simulink model "bipedal_robot_CTRL2"  (R2020b)
settings: Solver=ode23  StartTime=0.0  StopTime=Tsim  MaxStep=0.01  RelTol=1e-3  AbsTol=1e-3  EnableMultiTasking=on
values from neighbouring files (symbols this model uses):
  g = 9.80665    [bipedal.m]
  Tfil = Ts*10    (= 0.01)    [bipedal.m]
  total_mass = mlist(1) + ll_mass + rl_mass    [bipedal.m]
  Ts = 1/fs    (= 0.001)    [bipedal.m]
undefined symbols (not defined in the file or in its folder): Base, ctrl_cfg_rem, Fdist, LefAnklePitch, LefAnkleRoll, LefHipPitch, LefHipRoll, LefHipYaw, LefKnee, pg_traj, RigAnklePitch, RigAnkleRoll, RigHipPitch, RigHipRoll, RigHipYaw, RigKnee, sim_floor, Tdist, VAR_DIST, X, Y, Z
libraries: sm_lib x56, biped_lib x39, nesl_utility x18, simulink x3, Contact_Forces_Lib x2, robotmaniplib x1
(part 4 of 4)

== matlab function bipedal_robot_CTRL2/Controller Version 2/Compute torques/Error computation ==
  data: ctrl_cfg input; q_ref input; qp_ref input; qL input; errL output; qR input; errR output; errL_p output; errR_p output; intL output; intR output; qLp input; qRp input
function [errL, errR, errL_p, errR_p, intL, intR] = fcn(ctrl_cfg, q_ref, qp_ref, qL, qR, qLp, qRp)
persistent init errL_int errR_int;
if isempty(init)
   init = 1;
   errL_int = zeros(6,1);
   errR_int = zeros(6,1);
end

dt = ctrl_cfg.par.Ts;

% reference positions
qL_ref = q_ref(1:end/2);
qR_ref = q_ref(end/2+1:end);
% reference velocities
qLp_ref = qp_ref(1:end/2);
qRp_ref = qp_ref(end/2+1:end);


% measured positions
qL_m = qL;
qR_m = qR;
% measured velocities
qLp_m = qLp;
qRp_m = qRp;

% position errors
errL = qL_ref-qL_m;
errR = qR_ref-qR_m;

% integral term
errL_int = errL_int + dt * errL;
intL = errL_int;
errR_int = errR_int + dt * errR;
intR = errR_int;

% velocity errors
errL_p = qLp_ref-qLp_m;
errR_p = qRp_ref-qRp_m;

== matlab function bipedal_robot_CTRL2/Controller Version 2/Inverse kinematics optimization/Fmincon Ikine (Matlab)/Full body IKine solver ==
  data: FSM input; ctrl_cfg input; meas input; q_ref output; cmds input; Jlist input; phase input; cont_data input; qp_ref output; q_ini input; qp_ini input; FmL input; FmR input
function [q_ref,qp_ref] = fcn(FSM, ctrl_cfg, meas, cmds, Jlist, phase, cont_data, q_ini, qp_ini, FmL,FmR)
% check if ikine is activated
if FSM.ikine
    test_type = ctrl_cfg.fsm.test_type;
    
    if test_type==-1
        [q_ref,qp_ref] = ikine_step_iktest(meas, cmds, q_ini, qp_ini, Jlist, ctrl_cfg, phase, cont_data);
    else
        [q_ref,qp_ref] = ikine_step2(meas, cmds, q_ini, qp_ini, Jlist, ctrl_cfg, phase, cont_data);
    end
    
    active_FT_ctrl = 0;
    Ts = ctrl_cfg.par.Ts;
    [q_ref,qp_ref] = foot_tilt_ctrl2(FmL, FmR, q_ref, qp_ref, Ts, active_FT_ctrl);
    
    
else
    q_ref = q_ini;
    qp_ref = qp_ini;
end

== matlab function bipedal_robot_CTRL2/Controller Version 2/Finite state machine ==
  data: time input; FSM output Bus: FSM_bus; ctrl_cfg input; Ffil input; cont_data input; phase_data input; wGain output
function [FSM,wGain] = fcn(time, ctrl_cfg, Ffil, cont_data, phase_data)
    persistent fsm_state Tstart Tend dTst fsm_init;
    if isempty(fsm_state)
        fsm_state = 0;
        fsm_init = 1;
        Tstart = 0;
        Tend = 0;
        dTst = 0;
    end

    FL = Ffil(1);
    FR = Ffil(2);
    %stL = cont_data.L.state;
    %stR = cont_data.R.state;
    phase = phase_data.phase;
    wShiftL = phase_data.w(1);
    wShiftR = phase_data.w(2);


    test_type = ctrl_cfg.fsm.test_type;
    Tpause = ctrl_cfg.fsm.Tpause;

    FSM = fsm_ctrl_struct;
    %FSM.bal.act = 1;
    %FSM.bal.type = 1;
    % wait for the fb estimation to get the correct state
    FSM.bal.type = 2;



    if time >= Tpause
        if FSM.bal.type == 3
            FSM.gs.reduce_gains = 1;
        end

        if test_type == -1
            FSM.bal.act = 0;
            FSM.ikine = 1;
            FSM.pg_act = 1;
            FSM.tg.act = 0;
        elseif test_type == 0
            FSM.bal.act = 1;
            FSM.ikine = 1;
            FSM.pg_act = 0;
            FSM.tg.act = 0;
        else 
            FSM.bal.act = 1;
            FSM.ikine = 1;
            FSM.pg_act = 1;
            FSM.tg.act = 1;
        end
    end

    if fsm_init
        if fsm_state == 0
            dTst = ctrl_cfg.fsm.Tpause;
        elseif fsm_state == 1
            dTst = ctrl_cfg.fsm.times.Tini + ctrl_cfg.fsm.times.Tds/2;
        elseif fsm_state == 2 || fsm_state == 4
            dTst = ctrl_cfg.fsm.times.Tss;
        elseif fsm_state == 3 || fsm_state == 5
            dTst = ctrl_cfg.fsm.times.Tds;
        else
            dTst = ctrl_cfg.fsm.times.Tds/2 + ctrl_cfg.fsm.times.Tfin;
        end

        if fsm_state == 0
            Tstart = 0;
            Tend = dTst;
        else
            Tstart = Tend;
            Tend = Tend + dTst;
        end
        fsm_init = 0;
    end

    %time always starts from 0
    Tph = time - Tstart;

    Qtr_st = 0.5;
    Qtr_en = 0.9;

    trans_crit = 1;
    wGain = [0;0];
     %% finite state machine
    if fsm_state == 0
        %starting phase
        fsm_state_next = 1; %go to init DS

    elseif fsm_state == 1
        %initial DS phase
        if wShiftL>wShiftR
            fsm_state_next = 2; %go to left SS
        else
            fsm_state_next = 4; %go to right SS
        end

        if Tph > dTst*Qtr_en
            %one of the feet needs to transition into SS
            wGainS = gainWeight(dTst, Qtr_en, Tph,1);
            if fsm_state_next==2
                wGain(2) = wGainS;
            else
                wGain(1) = wGainS;
            end
        end

    elseif fsm_state == 6
        fsm_state_next = 6;
    else
        if fsm_state == 2 || fsm_state == 4
            % SS phase
            if fsm_state == 2
                % SS: left foot is the support one
                wGain(2) = 1;
                fsm_state_next = 3;
            else %if fsm_state == 4
                % right foot is the support one
                wGain(1) = 1;
                fsm_state_next = 5;
            end
        else

            if Tph < dTst*Qtr_st
                % foot needs to transition into DS
                wGainS = 1 - gainWeight(dTst, Qtr_st, Tph, 0);
                trType = 1;
            elseif Tph > dTst*Qtr_en
                % foot needs to transition into SS
                wGainS = gainWeight(dTst, Qtr_en, Tph, 1);
                trType = 2;
            else
                wGainS = 0;
                trType = 0;
            end

            if fsm_state == 3
                % DS: shifting weight from left to right
                if trType==1
                    wGain(2) = wGainS; %right foot into DS
                elseif trType==2
                    wGain(1) = wGainS; %left foot into SS
                end
                fsm_state_next = 4;

            else %if fsm_state == 5   
                % DS: shifting weight from right to left
                if trType==1
                    wGain(1) = wGainS; %left foot into DS
                elseif trType==2
                    wGain(2) = wGainS; %right foot into SS
                end
                fsm_state_next = 2;
            end
        end
    end

    if trans_crit && time>=Tend
        fsm_state = fsm_state_next;
        fsm_init = 1;
    end

    
end

== matlab function bipedal_robot_CTRL2/MATLAB Function ==
  data: Hb_eeL output; Hb_eeR output; tfb input; Hw_b output; Rfb input; MSL input; MSR input; qL output; qR output
function [Hb_eeL, Hb_eeR, Hw_b, qL, qR] = fcn(tfb, Rfb, MSL, MSR)
Hw_b = [Rfb,tfb;zeros(1,3),1];
[LL,RL] = group_motor_data(MSL,MSR);
qL = LL.q;
qR = RL.q;
Hb_L= H_abs_bL(qL);
Hb_R= H_abs_bR(qR);
Hb_eeL = reshape(Hb_L(end,:,:),4,4);
Hb_eeR = reshape(Hb_R(end,:,:),4,4);

== matlab function bipedal_robot_CTRL2/Controller Version 2/Compute torques/Group data ==
  data: MSL input; qL output; MSR input; qR output; qLp output; qRp output
function [qL,qR,qLp,qRp] = fcn(MSL, MSR)
% measurement data
[LL,RL] = group_motor_data(MSL,MSR);
qL = LL.q;
qLp = LL.qp;
qR = RL.q;
qRp = RL.qp;

== matlab function bipedal_robot_CTRL2/Controller Version 2/Pattern Generation/Pattern Generator ==
  data: FSM input; zmp output; time input; ctrl_cfg input; w output; targs output; phase output; pg_traj input
function [zmp,w,targs,phase]  = fcn(FSM, time, ctrl_cfg, pg_traj)
persistent t0;

traj = pg_traj;
Ts = ctrl_cfg.par.Ts;

if isempty(t0)
    t0 = time;
end

if ~FSM.pg_act
    %reset the time
    t0 = time;
    %output the zero values
    zmp = traj.zmp(:,1);
    w = traj.w(:,1);
    targs = [
        traj.foot.xL(:,1);
        traj.foot.xR(:,1);
        traj.foot.xLp(:,1);
        traj.foot.xRp(:,1);
    ];
    phase = traj.phase(1);
else
    t1 = time - t0;
    ii = round(t1/Ts);
    zmp = traj.zmp(:,ii);
    w = traj.w(:,ii);
    targs = [
        traj.foot.xL(:,ii);
        traj.foot.xR(:,ii);
        traj.foot.xLp(:,ii);
        traj.foot.xRp(:,ii);
    ];
    phase = traj.phase(ii);
end

== matlab function bipedal_robot_CTRL2/Controller Version 2/Trajectory Generation/Preview Controller (simulink impl)/MATLAB Function ==
  data: FSM input; reset output; use_meas output
function [reset,use_meas] = fcn(FSM)
% flush buffer memory
if ~FSM.tg.act
    reset = 1;
else
    reset = 0;
end

% use feedback (measured COM)
if FSM.tg.use_fb
    use_meas = 1;
else
    use_meas = 0;
end

== matlab function bipedal_robot_CTRL2/Controller Version 2/State Estimation/Fkine ==
  data: MSL input; Hb_L output; Hb_eeL output; MSR input; Hb_R output; Hb_eeR output; Hb_comi output; qLm output; qRm output
function [Hb_L, Hb_eeL, Hb_R, Hb_eeR, Hb_comi, qLm, qRm] = fcn(MSL,MSR)
    [LL,RL] = group_motor_data(MSL,MSR);
    qLm = LL.q;
    qRm = RL.q;
    [Hb_comi,Hb_L,Hb_R] = H_com_list(qLm,qRm);
    Hb_eeL = reshape(Hb_L(end,:,:),4,4);
    Hb_eeR = reshape(Hb_R(end,:,:),4,4);
end

== matlab function bipedal_robot_CTRL2/Controller Version 2/State Estimation/Floating base estimation ==
  data: FSM input; ctrl_cfg input; phase_data input; Hb_eeL input; Hw_b output; Hb_eeR input; MSL input; MSR input; FSL input; FSR input; tw_b output
function [Hw_b, tw_b] = fcn(FSM, ctrl_cfg, phase_data, Hb_eeL, Hb_eeR, MSL, MSR, FSL, FSR)
    persistent init Hw_L_corr Hw_R_corr;
    persistent quatLimu_old quatRimu_old;
    
    fb_est = ctrl_cfg.fb_est;
    cdf_data = fb_est.cdf_data;
    FootDataPmeas = fb_est.foot_data.fsen.Pmeas;
    
    phase = phase_data.phase;
    wsL = phase_data.w(1);
    wsR = phase_data.w(2);

    %begin by not doing any compensation (IMU has no bias yet)
    if isempty(init)
        %initialise persistent variables
        init = 1;
        Hw_L_corr = eye(4);
        Hw_R_corr = eye(4);
        quatLimu_old = [1;0;0;0];
        quatRimu_old = quatLimu_old;

        %only executed at the init phase
        Hw_eeL = fb_est.init.Hw_eeL;
        Hw_eeR = fb_est.init.Hw_eeR;
    else
        %if the drift compensation is activated, this is executed every time
        Hw_eeL = Hw_L_corr;
        Hw_eeR = Hw_R_corr;
    end

    %% Measurements from motors
    [LL,RL] = group_motor_data(MSL,MSR);
    aL = LL.a;
    aR = RL.a;
    wL = LL.w;
    wR = RL.w;

    %% IMU based rotation estimation
    %two imu-s that are rigidly attached to the floating base
    R_b_imu1L = rotz(-pi/6);
    R_b_imu1R = rotz(+pi/6);

    %measurements from those two imus
    a1Limu = aL(:,1);
    a1Rimu = aR(:,1);
    w1Limu = wL(:,1);
    w1Rimu = wR(:,1);

    %represent measurements in the base frame (just allignment, not spatial
    %transformation - this means, that we are still working with the
    %acceleration experienced at the position of the IMU)
    a1Lb = R_b_imu1L*a1Limu;
    a1Rb = R_b_imu1R*a1Rimu;
    w1Lb = R_b_imu1L*w1Limu;
    w1Rb = R_b_imu1R*w1Rimu;

    %sampling rate
    dt = fb_est.Ts;
    %use the magdwick algorithm to obtain the estimated rotation in the wcf
    %left
    quatLimu = filter_update(a1Lb, w1Lb, quatLimu_old);
    quatLimu_old = quatLimu;

    %right
    quatRimu = filter_update(a1Rb, w1Rb, quatRimu_old);
    quatRimu_old = quatRimu; 

    %measurements can not be merged directly, as they were obtained in
    %different frames. Calculated quaternions however can be merged, as they
    %are representing the rotation of the same body.
    %averaging rotation matrices - Henze and Ott - documented in 3.2 FB pose
    %est.
    quat_imu_sum = (quatLimu+quatRimu)/2;
    quat_imu_merged = quat_imu_sum/norm(quat_imu_sum); %orientation from the accelerometer
    Rw_b_imu = quat2rotm(quat_imu_merged');

    %% kinematics based rotation estimation
    %translations which are needed for later
    pb_eeL = Hb_eeL(1:3,4);
    pb_eeR = Hb_eeR(1:3,4);

    %kinematic guess for the transformation between wcf and base 
    Hw_b_Lleg = Hw_eeL/Hb_eeL;
    Hw_b_Rleg = Hw_eeR/Hb_eeR;

    %rotations
    Rw_b_Lleg = Hw_b_Lleg(1:3,1:3);
    Rw_b_Rleg = Hw_b_Rleg(1:3,1:3);
    %translations
    pw_b_Lleg = Hw_b_Lleg(1:3,4);
    pw_b_Rleg = Hw_b_Rleg(1:3,4);

    %% fuse all three measurements depending on the leg ZMP measurements
    %flight leg is assigned a low weight, whereas stance leg obtains a high one
    %the closet the zmp is to the edge, the lower the weight is
    zmp_cdf = cdf_data.zmp;
    fcont_cdf = cdf_data.cont;

    %compute the values based on the model and force measurements (LFL&LFR)
    [zmpL] = compute_local_zmp_simple(FSL.Fm,FootDataPmeas);
    [zmpR] = compute_local_zmp_simple(FSR.Fm,FootDataPmeas);
    ftot_L = sum(FSL.Fm);
    ftot_R = sum(FSR.Fm);

    %compute weights
    WL_zmp = max(0,interp2(zmp_cdf.x,zmp_cdf.y,zmp_cdf.p,zmpL(1),zmpL(2)));
    WL_cont = min(max(0,interp1(fcont_cdf.f,fcont_cdf.p,ftot_L,'linear','extrap')),1);

    WR_zmp = max(0,interp2(zmp_cdf.x,zmp_cdf.y,zmp_cdf.p,zmpR(2),zmpR(2)));
    WR_cont = min(max(0,interp1(fcont_cdf.f,fcont_cdf.p,ftot_R,'linear','extrap')),1);

    %single support phase
%     if phase==1
%         if wsL>wsR
%             %right is the flight foot
%             WR_zmp = 0;
%             WR_cont = 0;
%         else
%             %left is the flight foot
%             WL_zmp = 0;
%             WL_cont = 0;
%         end
%     end

    %kinematic weights depend on contact estimation and zmp trust region
    WL = WL_zmp*WL_cont;
    WR = WR_zmp*WR_cont;
    Wimu = 0.1;

    eps = 1e-12;
    %normalise weights
    W_norm1 = 1/(WR+WL+eps);
    W_norm2 = 1/(Wimu+WR+WL+eps);
    Wimu_vec = Wimu * [0, W_norm2, W_norm2]; %discard the first angle which is yaw (ZYX convention)
    WL_vec = WL * [W_norm1, W_norm2, W_norm2];
    WR_vec = WR * [W_norm1, W_norm2, W_norm2];

    %fuse measurements using the computed weights
    eul_fused = Wimu_vec.*rotm2eul(Rw_b_imu) + WL_vec.*rotm2eul(Rw_b_Lleg) + WR_vec.*rotm2eul(Rw_b_Rleg);
    Rest_w_b = eul2rotm(eul_fused);

    %% compute the position of the fb in the wcf (averaging two feet)
    pest_w_b = (WL*(Hw_eeL(1:3,4)-Rest_w_b*pb_eeL)+WR*(Hw_eeR(1:3,4)-Rest_w_b*pb_eeR)) * W_norm1;

    %% generate the Hwb transformation and compensate for drifts
    Hest_w_b = [
        Rest_w_b,pest_w_b;
        zeros(1,3),1;
    ];

    %compute drift transformations
    HLdrift = Hw_eeL\Hest_w_b*Hb_eeL;
    HRdrift = Hw_eeR\Hest_w_b*Hb_eeR;

    %compensation factor (between 0 [no convg] and 1 [full comp]) - has to be
    %tuned
    alpha = fb_est.alpha; 
    %it is correct that left and right side are inverted, as stance foot will
    %not drift, however it determines how much the swing foot will
    alphaL = alpha*WR;
    alphaR = alpha*WL;
    [HcorrL,~,~] = transformtraj(eye(4),HLdrift,[0 1],alphaL);
    [HcorrR,~,~] = transformtraj(eye(4),HRdrift,[0 1],alphaR);
    Hw_L_corr = Hw_eeL*HcorrL;
    Hw_R_corr = Hw_eeR*HcorrR;

    Hw_b = Hest_w_b;
    tw_b = pest_w_b;
end

== matlab function bipedal_robot_CTRL2/Controller Version 2/Balancer ==
  data: x_com output; FSM input; ctrl_cfg input; tg_data input; xp_com output; fb_est_data input; TL output; TR output; phase_data input; Hw_b input; Hb_c input; jacobian input
function [x_com,xp_com,TL,TR] = fcn(FSM, ctrl_cfg, tg_data, fb_est_data, phase_data, Hw_b, Hb_c, jacobian)
    persistent init dcm_int comz_int x_com_old v_com_old;
    if isempty(init)
        init = 1;
        dcm_int = zeros(2,1);
        comz_int = 0;
        v_com_old = zeros(3,1);
        x_com_old = [0;0;ctrl_cfg.bal.com_height];
    end


    %% data about support
    w = phase_data.w;
    WshiftL = w(1);
    WshiftR = w(2);
    phase = phase_data.phase;
    
    %% jacobians
    Jb_eeL = jacobian.Jb_eeL;
    Jb_eeR = jacobian.Jb_eeR;

    %% constants & configuration
    Ts = ctrl_cfg.par.Ts;
    z_des = ctrl_cfg.bal.com_height;
    g = 9.81;
    omega = sqrt(g/z_des);
    mlist = ctrl_cfg.bal.mlist;
    Mtot = sum(mlist);
    foot_data = ctrl_cfg.bal.foot_data;
    foot_dims = foot_data.dims(1:2)*0.9;
    K = Mtot*omega^2;

    %% read measurements
    zmp_m = fb_est_data.zmp;
    com_m = fb_est_data.com;
    comp_m = fb_est_data.comp;
    dcm_m = fb_est_data.dcm; 
    Hb_eeL = fb_est_data.Hb_eeL;
    Hb_eeR = fb_est_data.Hb_eeR;

    %% read controls
    zmp_d = tg_data.zmp;
    com_d = tg_data.com;
    comp_d = tg_data.comp;
    dcm_d = tg_data.dcm;
    dcmp_d = tg_data.dcmp;
    
    TL = zeros(6,1);
    TR = zeros(6,1);
    v_com = zeros(3,1);
    % check if the stabilisation is activated
    if FSM.bal.act
        %% controller possibility 1
        if FSM.bal.type == 1
            % gains
            Kp_dcm = [1.6*omega;1.3*omega];
            Kp_comz = 3000*omega;
            Kd_comz = 800*omega;
            Ki_comz = 3000*omega;
            Kp_zmp = [0.2*omega;0.2*omega];
            % leaky integrator
            Ki_dcm = [1*omega;1*omega];
            Kleak = [0.1;0.1];


            % controller
            % com-z
            comz_err = com_d(3) - com_m(3);
            comz_int = comz_int + Ts * comz_err;
            comzpp_r = Kd_comz*(comp_d(3)-comp_m(3)) + Kp_comz*comz_err + Ki_comz*comz_int;

            % dcm integrator
            dcm_err = dcm_d(1:2) - dcm_m(1:2); %integral error
            d_err = dcm_err - Kleak.*dcm_int; %inclusion of leakage
            dcm_int = dcm_int + Ts * d_err;

            % reference value for the ZMP
            zmp_r = zmp_d -(1+Kp_dcm./omega).*dcm_err - Ki_dcm./omega.*dcm_int + Kp_zmp./omega.*(zmp_d-zmp_m);

            % force
            Admittance = eye(3)*0.1;
            Fd = [
                K*(com_m(1)-zmp_r(1));
                K*(com_m(2)-zmp_r(2));
                comzpp_r;
            ];

            a_com = Admittance * Fd/Mtot;
            v_com = v_com_old + a_com * Ts; 
            v_com_old = v_com;
            

        %% controller possibility 2
        elseif FSM.bal.type == 2
            % gains
            Kp_dcm = [1;1];
            Kp_comz = 0;
            Ki_comz = 0;
            Kp_zmp = [0.7;0.5]*omega;
            K_com = [4.0;5.0]*omega;
            % leaky integrator
            Ki_dcm = [0;0];
            Kleak = [0.1;0.1];
            
            % controller
            % com-z
            comz_err = com_d(3) - com_m(3);
            comz_int = comz_int + Ts * comz_err;
            comzp_r = comp_d(3) + Kp_comz*comz_err + Ki_comz*comz_int;
            
            % dcm integrator
            dcm_err = dcm_d(1:2) - dcm_m(1:2); %integral error
            d_err = dcm_err - Kleak.*dcm_int; %inclusion of leakage
            dcm_int = dcm_int + Ts * d_err;
            
            zmp_r = dcm_d(1:2) - dcmp_d(1:2)/omega + Kp_dcm .* d_err + Ki_dcm .* dcm_int;
            
            v_com = [
                comp_d(1:2) - Kp_zmp .* (zmp_r - zmp_m) + K_com .* (com_d(1:2) - com_m(1:2));
                0;
            ];
        
        else    
             % gains
%             Kp_dcm = [1.6;1.5];
%             Kp_comz = 30*omega;
%             Kd_comz = 8*omega;
%             Ki_comz = 0;
%             Kp_zmp = [0.5;0.5]*omega;
%             K_com = [1.5;1.5]*omega;
%             % leaky integrator
%             Ki_dcm = [1;1]*0;
%             Kleak = [0.1;0.1];
%             
%             % controller
%             % com-z
%             comz_err = com_d(3) - com_m(3);
%             comz_int = comz_int + Ts * comz_err;
%             comzpp_r = Kd_comz*(comp_d(3)-comp_m(3)) + Kp_comz*comz_err + Ki_comz*comz_int;
%             
%             % dcm integrator
%             dcm_err = dcm_d(1:2) - dcm_m(1:2); %integral error
%             d_err = dcm_err - Kleak.*dcm_int; %inclusion of leakage
%             dcm_int = dcm_int + Ts * d_err;
%             
%             zmp_r = dcm_d(1:2) - dcmp_d(1:2)/omega + Kp_dcm .* d_err + Ki_dcm .* dcm_int;
%             
%             
%             
%             Wc = [0;0;-(Mtot*g+comzpp_r);0;0;0];
%             Hc_b = inv(Hb_c);
%             [Wlfoot,Wrfoot] = distribute_wrench_tracking(Wc,Jb_eeL,Jb_eeR,Hc_b,Hb_eeL,Hb_eeR,foot_dims,0.6,0,phase,WshiftL,WshiftR);
%             
%             v_com = [
%                 comp_d(1:2) - Kp_zmp .* (zmp_r - zmp_m) + K_com .* (com_d(1:2) - com_m(1:2));
%                 0;
%             ];
%         
%             %gravity compensation
%             TL = Jb_eeL'*Wlfoot;
%             TR = Jb_eeR'*Wrfoot;
        end
    else
        v_com = zeros(3,1);
    end
    
    x_com = x_com_old + v_com * Ts; 
    x_com_old = x_com;
    
    xp_com = v_com;
